simulink model "model_dynamika"  (R2014b)
settings: Solver=ode23  StartTime=0.0  StopTime=15.0  RelTol=1e-10
values from neighbouring files (symbols this model uses):
  K = 100    [dynamika.m]    (also in monocykl.m)
  k1 = 1    [dynamika.m]    (also in kinematyka.m; monocykl.m)
  k2 = 1    [dynamika.m]    (also in kinematyka.m; monocykl.m)
  M11 = Mc+2*Mk*L*L    (= 107.9)    [dynamika.m]    (also in monocykl.m; wielomianowy.m)
  M22 = Ip/(L*L)    (= 83.5895833333)    [dynamika.m]    (also in monocykl.m; wielomianowy.m)
  R = 5    [dynamika.m]    (also in kinematyka.m)
  teta0 = 0    [dynamika.m]    (also in kinematyka.m; monocykl.m = 3; wielomianowy.m)
  w = 1    [dynamika.m]    (also in kinematyka.m)
  x0 = 0    [dynamika.m]    (also in kinematyka.m; monocykl.m = 4; wielomianowy.m = 1)
  y0 = 0    [dynamika.m]    (also in kinematyka.m; monocykl.m = 2; wielomianowy.m = 2)
settings Model: Creator=lab1.5  LastModifiedBy=Dawid Perdek

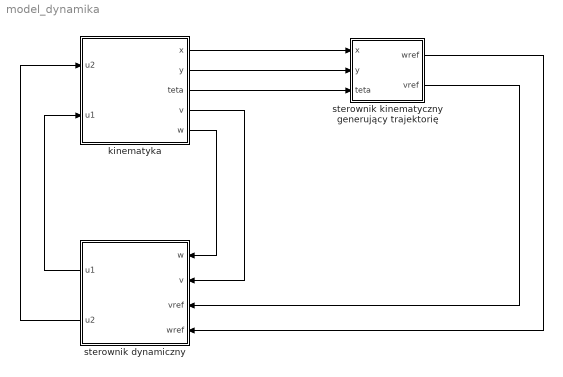
== system model_dynamika ==
  kinematyka : Subsystem
  sterownik dynamiczny : Subsystem
  sterownik kinematyczny generujący trajektorię : Subsystem
  wires:
  kinematyka/1(x) -> sterownik kinematyczny generujący trajektorię/1(x)
  kinematyka/2(y) -> sterownik kinematyczny generujący trajektorię/2(y)
  kinematyka/3(teta) -> sterownik kinematyczny generujący trajektorię/3(teta)
  sterownik kinematyczny generujący trajektorię/1(wref) -> sterownik dynamiczny/4(wref)
  sterownik kinematyczny generujący trajektorię/2(vref) -> sterownik dynamiczny/3(vref)
  sterownik dynamiczny/1(u1) -> kinematyka/2(u1)
  sterownik dynamiczny/2(u2) -> kinematyka/1(u2)
  kinematyka/5(w) -> sterownik dynamiczny/1(w)
  kinematyka/4(v) -> sterownik dynamiczny/2(v)

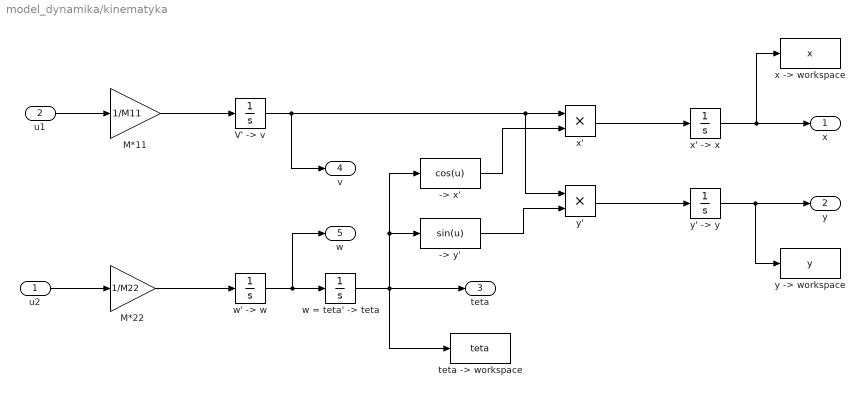
== system model_dynamika/kinematyka ==
  u2 : Inport
  u1 : Inport  Port=2
  -> x' : Fcn  Expr=cos(u)
  -> y' : Fcn  Expr=sin(u)
  M*11 : Gain  Gain=1/M11
  M*22 : Gain  Gain=1/M22
  "V' -> v" : Integrator
  "teta -> workspace" : ToWorkspace  VariableName=teta  SampleTime=-1
  "w = teta' -> teta" : Integrator  InitialCondition=teta0
  "w' -> w" : Integrator
  "x -> workspace" : ToWorkspace  VariableName=x  SampleTime=-1
  x' : Product
  "x' -> x" : Integrator  InitialCondition=x0
  "y -> workspace" : ToWorkspace  VariableName=y  SampleTime=-1
  y' : Product
  "y' -> y" : Integrator  InitialCondition=y0
  x : Outport
  y : Outport  Port=2
  teta : Outport  Port=3
  v : Outport  Port=4
  w : Outport  Port=5
  wires:
  u2/1 -> M*22/1
  u1/1 -> M*11/1
  -> x'/1 -> x'/2
  -> y'/1 -> y'/2
  x'/1 -> "x' -> x"/1
  y'/1 -> "y' -> y"/1
  "x' -> x"/1 -> "x -> workspace"/1, x/1
  "y' -> y"/1 -> "y -> workspace"/1, y/1
  "w = teta' -> teta"/1 -> "teta -> workspace"/1, -> x'/1, -> y'/1, teta/1
  M*11/1 -> "V' -> v"/1
  "V' -> v"/1 -> v/1, y'/1, x'/1
  M*22/1 -> "w' -> w"/1
  "w' -> w"/1 -> w/1, "w = teta' -> teta"/1

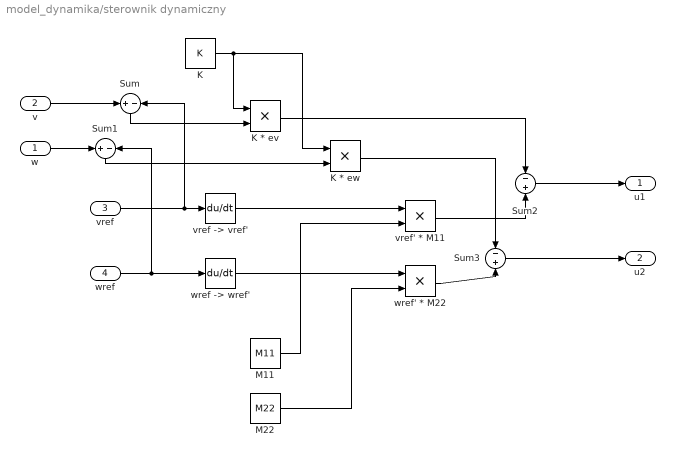
== system model_dynamika/sterownik dynamiczny ==
  w : Inport
  v : Inport  Port=2
  vref : Inport  Port=3
  wref : Inport  Port=4
  K : Constant  Value=K
  K * ev : Product
  K * ew : Product
  M11 : Constant  Value=M11
  M22 : Constant  Value=M22
  Sum : Sum  Inputs=+-
  Sum1 : Sum  Inputs=+-
  Sum2 : Sum  Inputs=-+
  Sum3 : Sum  Inputs=-+
  "vref -> vref'" : Derivative
  vref' * M11 : Product
  "wref -> wref'" : Derivative
  wref' * M22 : Product
  u1 : Outport
  u2 : Outport  Port=2
  wires:
  vref/1 -> Sum/2, "vref -> vref'"/1
  wref/1 -> Sum1/2, "wref -> wref'"/1
  "vref -> vref'"/1 -> vref' * M11/1
  M11/1 -> vref' * M11/2
  "wref -> wref'"/1 -> wref' * M22/1
  M22/1 -> wref' * M22/2
  v/1 -> Sum/1
  w/1 -> Sum1/1
  Sum/1 -> K * ev/2
  Sum1/1 -> K * ew/2
  K/1 -> K * ew/1, K * ev/1
  vref' * M11/1 -> Sum2/2
  K * ev/1 -> Sum2/1
  wref' * M22/1 -> Sum3/2
  K * ew/1 -> Sum3/1
  Sum2/1 -> u1/1
  Sum3/1 -> u2/1

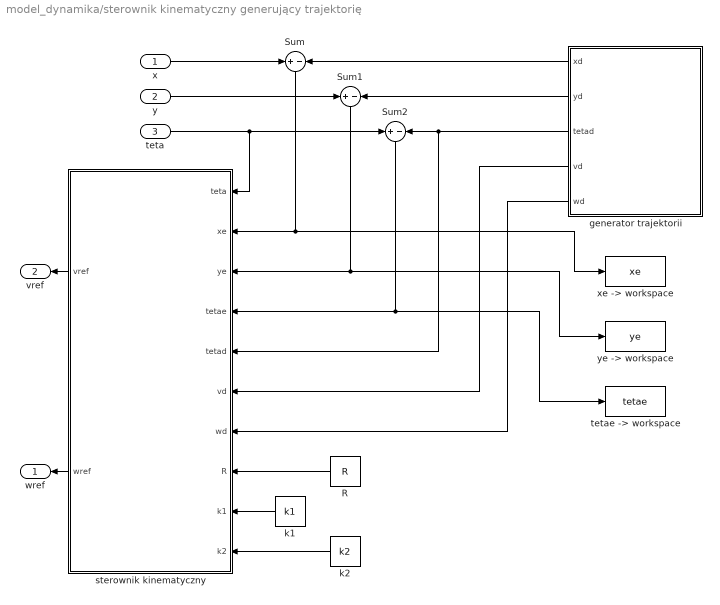
== system model_dynamika/sterownik kinematyczny generujący trajektorię ==
  x : Inport
  y : Inport  Port=2
  teta : Inport  Port=3
  R : Constant  Value=R
  Sum : Sum  Inputs=+-
  Sum1 : Sum  Inputs=+-
  Sum2 : Sum  Inputs=+-
  generator trajektorii : Subsystem
  k1 : Constant  Value=k1
  k2 : Constant  Value=k2
  sterownik kinematyczny : MATLAB Function  TreatAsAtomicUnit=on
  "tetae -> workspace" : ToWorkspace  VariableName=tetae  SampleTime=-1
  "xe -> workspace" : ToWorkspace  VariableName=xe  SampleTime=-1
  "ye -> workspace" : ToWorkspace  VariableName=ye  SampleTime=-1
  wref : Outport
  vref : Outport  Port=2
  wires:
  sterownik kinematyczny/1(vref) -> vref/1
  sterownik kinematyczny/2(wref) -> wref/1
  x/1 -> Sum/1
  y/1 -> Sum1/1
  teta/1 -> sterownik kinematyczny/1(teta), Sum2/1
  generator trajektorii/1(xd) -> Sum/2
  generator trajektorii/2(yd) -> Sum1/2
  generator trajektorii/3(tetad) -> sterownik kinematyczny/5(tetad), Sum2/2
  k1/1 -> sterownik kinematyczny/9(k1)
  k2/1 -> sterownik kinematyczny/10(k2)
  R/1 -> sterownik kinematyczny/8(R)
  Sum/1 -> sterownik kinematyczny/2(xe), "xe -> workspace"/1
  Sum1/1 -> "ye -> workspace"/1, sterownik kinematyczny/3(ye)
  Sum2/1 -> sterownik kinematyczny/4(tetae), "tetae -> workspace"/1
  generator trajektorii/4(vd) -> sterownik kinematyczny/6(vd)
  generator trajektorii/5(wd) -> sterownik kinematyczny/7(wd)

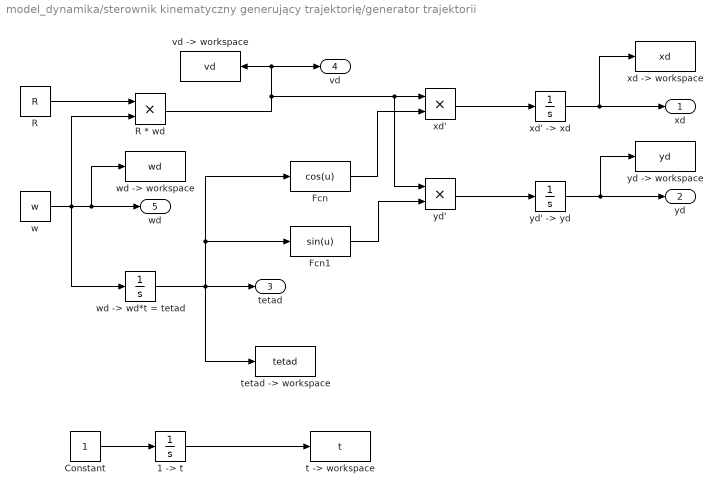
== system model_dynamika/sterownik kinematyczny generujący trajektorię/generator trajektorii ==
  "1 -> t" : Integrator
  Constant : Constant
  Fcn : Fcn  Expr=cos(u)
  Fcn1 : Fcn  Expr=sin(u)
  R : Constant  Value=R
  R * wd : Product
  "t -> workspace" : ToWorkspace  VariableName=t  SampleTime=-1
  "tetad -> workspace" : ToWorkspace  VariableName=tetad  SampleTime=-1
  "vd -> workspace" : ToWorkspace  VariableName=vd  SampleTime=-1
  w : Constant  Value=w
  "wd -> wd*t = tetad" : Integrator
  "wd -> workspace" : ToWorkspace  VariableName=wd  SampleTime=-1
  "xd -> workspace" : ToWorkspace  VariableName=xd  SampleTime=-1
  xd' : Product
  "xd' -> xd" : Integrator
  "yd -> workspace" : ToWorkspace  VariableName=yd  SampleTime=-1
  yd' : Product
  "yd' -> yd" : Integrator  InitialCondition=-R
  xd : Outport
  yd : Outport  Port=2
  tetad : Outport  Port=3
  vd : Outport  Port=4
  wd : Outport  Port=5
  wires:
  Constant/1 -> "1 -> t"/1
  "1 -> t"/1 -> "t -> workspace"/1
  w/1 -> "wd -> workspace"/1, wd/1, R * wd/2, "wd -> wd*t = tetad"/1
  "wd -> wd*t = tetad"/1 -> "tetad -> workspace"/1, tetad/1, Fcn/1, Fcn1/1
  R/1 -> R * wd/1
  R * wd/1 -> vd/1, "vd -> workspace"/1, yd'/1, xd'/1
  Fcn1/1 -> yd'/2
  Fcn/1 -> xd'/2
  "yd' -> yd"/1 -> yd/1, "yd -> workspace"/1
  xd'/1 -> "xd' -> xd"/1
  "xd' -> xd"/1 -> xd/1, "xd -> workspace"/1
  yd'/1 -> "yd' -> yd"/1

== matlab function model_dynamika/sterownik kinematyczny generujący trajektorię/sterownik kinematyczny ==
  data: teta input; xe input; ye input; tetae input; tetad input; vd input; wd input; R input; vref output; wref output; k1 input; k2 input
function [vref,wref] = sterownik_kinematyczny(teta,xe,ye,tetae,tetad,vd,wd,R,k1,k2)

ex = cos(teta) * xe + sin(teta) * ye;
ey = -sin(teta) * xe + cos(teta) * ye;
eteta = tetae;

w = tetad;
v = R*wd;

vref = vd * cos(eteta) - k1 * ex;
wref = wd - ey * vd - k2 * eteta;
